simulink model "ModeAdjust"  (R2018b)
settings: Solver=FixedStepDiscrete  StartTime=0.0  StopTime=inf  FixedStep=0.01  RelTol=1e-3
undefined symbols (not defined in the file or in its folder): IfKeSMSbSeatMovBkRclnEnable_Val, IfKeSMSbSeatMovFrwdBkwdEnable_Val, IfKeSMSbSeatMovFtrstEnable_Val, IfKeSMSbSeatMovHdrstFrwdBkwdEnable_Val, IfKeSMSbSeatMovHdUpwdDnwdEnable_Val, IfKeSMSbSeatMovLgrstEnable_Val, IfKeSMSbSeatMovLtwdRtwdEnable_Val, IfVeSMSeStNumConfig, KeSMSbArmscreenMovEnable_Val, KeSMSbSeatMovLgrstExpdEnable_Val, KeSMSuFirstRwStBackPosDelta_Val, KeSMSuFirstRwStBackPosTolr_Val, KeSMSuFirstRwStCushFrntPosDelta_Val, KeSMSuFirstRwStCushFrntPosTolr_Val, KeSMSuFirstRwStCushRePosDelta_Val, KeSMSuFirstRwStCushRePosTolr_Val, KeSMSuFirstRwStFootrestPosDelta_Val, KeSMSuFirstRwStFootrestPosTolr_Val, KeSMSuFirstRwStFwdBkwdPosDelta_Val, KeSMSuFirstRwStFwdBkwdPosTolr_Val, KeSMSuMdMotFinshdTm_Val, KeSMSuMdRetryTm1_Val, KeSMSuModeReqDurgTm_Val, KeSMSuSecRwStArmTochPosDelta_Val, KeSMSuSecRwStArmTochPosTolr_Val, KeSMSuSecRwStBackPosDelta_Val, KeSMSuSecRwStBackPosTolr_Val, KeSMSuSecRwStFtrstUpwdDnwdPosDelta_Val, KeSMSuSecRwStFtrstUpwdDnwdPosTolr_Val, KeSMSuSecRwStFwdBkwdPosDelta_Val, KeSMSuSecRwStFwdBkwdPosTolr_Val, KeSMSuSecRwStHeadrestFwdBkwdPosDelta_Val, KeSMSuSecRwStHeadrestFwdBkwdPosTolr_Val, KeSMSuSecRwStHeadrestUpwdDwnwdPosDelta_Val, KeSMSuSecRwStHeadrestUpwdDwnwdPosTolr_Val, KeSMSuSecRwStLegrestInOutPosDelta_Val, KeSMSuSecRwStLegrestInOutPosTolr_Val, KeSMSuSecRwStLegrestUpwdDwnwdPosDelta_Val, KeSMSuSecRwStLegrestUpwdDwnwdPosTolr_Val, KeSMSuSecRwStLwdRwdPosDelta_Val, KeSMSuSecRwStLwdRwdPosTolr_Val, KeSMSuSecRwStVIPFtrstRefAngle_Val, KeSMSuThirdRwStFwdBkwdPosDelta_Val, KeSMSuThirdRwStFwdBkwdPosTolr_Val, KeSMSuThrdRwCushFoldPosDelta_Val, KeSMSuThrdRwCushFoldPosTolr_Val, KeSMSuThrdRwStBackPosDelta_Val, KeSMSuThrdRwStBackPosTolr_Val, KeSMSw4SLegrstCloseMdSecRwLtStFtrstUpwdDnwdPos_Val, KeSMSw4SLegrstCloseMdSecRwLtStFtrstUpwdDnwdPosMax_Val, KeSMSw4SLegrstCloseMdSecRwLtStFtrstUpwdDnwdPosMin_Val, KeSMSw4SLegrstCloseMdSecRwLtStLgrstOtwdInwdPos_Val, KeSMSw4SLegrstCloseMdSecRwLtStLgrstOtwdInwdPosMax_Val, KeSMSw4SLegrstCloseMdSecRwLtStLgrstOtwdInwdPosMin_Val, KeSMSw4SLegrstCloseMdSecRwLtStLgrstUpwdDnwdPos_Val, KeSMSw4SLegrstCloseMdSecRwLtStLgrstUpwdDnwdPosMax_Val, KeSMSw4SLegrstCloseMdSecRwLtStLgrstUpwdDnwdPosMin_Val, KeSMSw4SLegrstCloseMdSecRwRtStFtrstUpwdDnwdPos_Val, KeSMSw4SLegrstCloseMdSecRwRtStFtrstUpwdDnwdPosMax_Val, KeSMSw4SLegrstCloseMdSecRwRtStFtrstUpwdDnwdPosMin_Val ... (+1138)
libraries: Lib x401
(part 21 of 35)

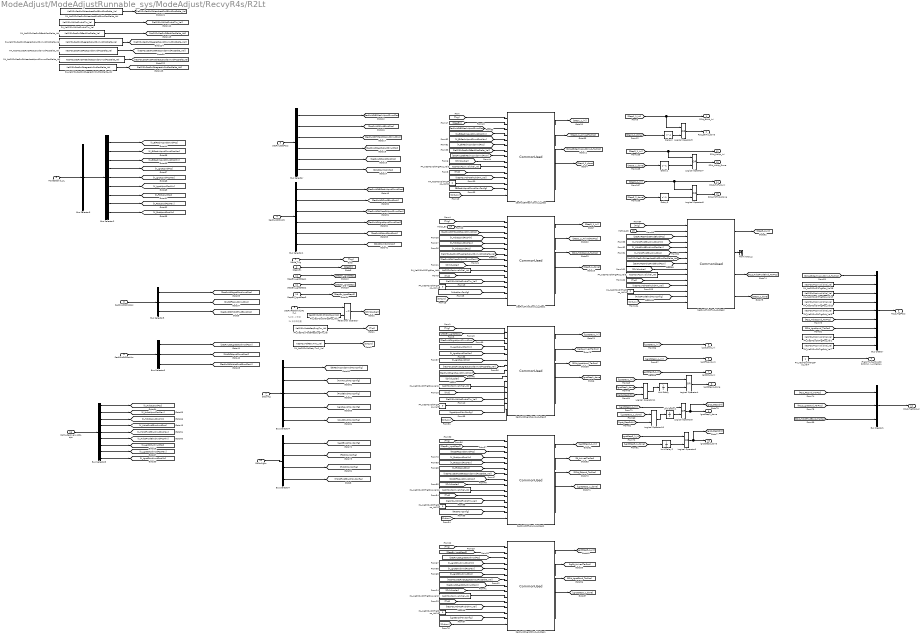
== system ModeAdjust/ModeAdjustRunnable_sys/ModeAdjust/RecvyR4s/R2Lt ==
  note: %1锁，2未锁
  note: 2L 扶手屏位置
  Mode_Trig : Inport
  Step1En : Inport  Port=2
  SecRwLtStsPoss : Inport  Port=3
  SecRwLtStPossV : Inport  Port=4
  SecRwRtStChldLkRsp_L : Inport  Port=5
  ModeStCalib_2L : Inport  Port=6
  StConfig : Inport  Port=7
  SecRwLtStsPoss4s : Inport  Port=8
  SecRwLtStPossV4s : Inport  Port=9
  StConfig4s : Inport  Port=10
  StepEn_LgrstStep1 : Inport  Port=11
  StepEn_LgrstStep2 : Inport  Port=12
  StepEn_LgrstStep3 : Inport  Port=13
  HdUp_En : Inport  Port=14
  HdFwd_En : Inport  Port=15
  Calib_Recovery4sRAdpt : Inport  Port=16
  Bus Creator : BusCreator  Inputs=9  OutDataTypeStr=Bus: SecRwRtSeatPos
  Bus Creator1 : BusCreator  Inputs=3
  Bus Selector : BusSelector  OutputSignals=IfVeSMSuSecRwRtStBkReclnUpwdDnwdPos_Val_read,IfVeSMSuSecRwRtStFrwdBkwdPos_Val_read,IfVeSMSuSecRwRtStHPassStUpwdDnwdPos_Val_read,IfVeSMSuSecRwRtStLgrstUpwdDnwdPos_Val_read,IfVeSMSuSecRwRtStLtwdRtwdPos_Val_read,SecRwRtStArmScrnPos_Val_read
  Bus Selector1 : BusSelector  OutputSignals=IfVeSMSuSecRwRtStBkReclnUpwdDnwdPosV_Val_read,IfVeSMSuSecRwRtStFrwdBkwdPosV_Val_read,IfVeSMSuSecRwRtStHPassStUpwdDnwdPosV_Val_read,IfVeSMSuSecRwRtStLgrstUpwdDnwdPosV_Val_read,IfVeSMSuSecRwRtStLtwdRtwdPosV_Val_read,SecRwRtStArmScrnPosV_Val_read
  Bus Selector2 : BusSelector  OutputSignals=BkReclnUpwdDnwdPos,BkReclnUpwdDnwdPosMax,BkReclnUpwdDnwdPosMin,LgrstUpwdPos,LgrstUpwdPosMax,LgrstUpwdPosMin,FtrstUpwdDnwdPos,FtrstUpwdDnwdPosMax,FtrstUpwdDnwdPosMin
  Bus Selector3 : BusSelector  OutputSignals=RecvyRSecRwRtSt
  Bus Selector4 : BusSelector  OutputSignals=BkReclnUpwdDnwdMovConfig,ArmTouchMovConfig,FrwdBkwdMovConfig,LgrstUpwdMovConfig,LtwdRtwdMovConfig
  Bus Selector5 : BusSelector  OutputSignals=IfVeSMSuSecRwRtStLgrstOtwdInwdPos_Val_read,IfVeSMSuRrRtStFtUpwdDnwdPos_Val_read,IfVeSMSuSecRwRtStHdrstFrwdBkwdPos_Val_read
  Bus Selector6 : BusSelector  OutputSignals=IfVeSMSuSecRwRtStLgrstOtwdInwdPosV_Val_read,IfVeSMSuRrRtStFtUpwdDnwdPosV_Val_read,IfVeSMSuSecRwRtStHdrstFrwdBkwdPosV_Val_read
  Bus Selector7 : BusSelector  OutputSignals=LgrstExpdMovConfig,FtrstMovConfig,HdrstUpwdDnwdMovConfig,HdrstFrwdBkwdMovConfig
  Bus Selector8 : BusSelector  OutputSignals=HdrstUpwdDnwdPos,HdrstUpwdDnwdPosMax,HdrstUpwdDnwdPosMin,HdrstFrwdBkwdnwdPos,HdrstFrwdBkwdnwdPosMax,HdrstFrwdBkwdnwdPosMin,LgrstOtwdInwdPos,LgrstOtwdInwdPosMax,LgrstOtwdInwdPosMin
  Delay1 : Delay  DelayLength=1
  Delay2 : Delay  DelayLength=1
  Delay3 : Delay  DelayLength=1
  Logical Operator10 : Logic  AllPortsSameDT=off  OutDataTypeStr=boolean
  Logical Operator11 : Logic  AllPortsSameDT=off  OutDataTypeStr=boolean
  Logical Operator{3..8} (6 alike) : Logic  Operator=OR  AllPortsSameDT=off  OutDataTypeStr=boolean
  PA_KeSMSuMdMotFinshdTm_Val : Constant  Value=KeSMSuMdMotFinshdTm_Val
  PA_KeSMSuMdRetryTm1_Val : Constant  Value=KeSMSuMdRetryTm1_Val
  PA_KeSMSuModeReqDurgTm_Val : Constant  Value=KeSMSuModeReqDurgTm_Val
  PA_KeSMSuSecRwStBackPosDelta_Val : Constant  Value=KeSMSuSecRwStBackPosDelta_Val
  PA_KeSMSuSecRwStFtrstUpwdDnwdPosDelta_Val : Constant  Value=KeSMSuSecRwStFtrstUpwdDnwdPosDelta_Val
  PA_KeSMSuSecRwStHeadrestFwdBkwdPosDelta_Val : Constant  Value=KeSMSuSecRwStHeadrestFwdBkwdPosDelta_Val
  PA_KeSMSuSecRwStHeadrestUpwdDwnwdPosDelta_Val : Constant  Value=KeSMSuSecRwStHeadrestUpwdDwnwdPosDelta_Val
  PA_KeSMSuSecRwStLegrestInOutPosDelta_Val : Constant  Value=KeSMSuSecRwStLegrestInOutPosDelta_Val
  PA_KeSMSuSecRwStLegrestUpwdDwnwdPosDelta_Val : Constant  Value=KeSMSuSecRwStLegrestUpwdDwnwdPosDelta_Val
  PA_KeSMSwDltTrgtPos_Val{1,3,5..8,12..13,16,18..20} (12 alike) : Constant  Value=KeSMSwPosInvalidVal_Val
  PA_KeSMSwDltTrgtPos_Val{9..11,15,22,30} (6 alike) : Constant  Value=0  OutDataTypeStr=boolean
  PA_KeSMSwDltTrgtPos_Val2 : Constant  Value=SeatChldLkSt.ChldLkSt_Unlock
  PA_KeSMSwDltTrgtPos_Val4 : Constant  OutDataTypeStr=boolean
  Relational Operator : RelationalOperator  Operator=~=  OutDataTypeStr=boolean  RndMeth=Simplest
  SecRwLtBkRecInUpwd_Lt_Step : Lib/CommonUsed  SystemSampleTime=-1
  SecRwLtHdrstFwd_Lt_Step2 : Lib/CommonUsed  SystemSampleTime=-1
  SecRwLtHdrstUpwd_Lt_Step1 : Lib/CommonUsed  SystemSampleTime=-1
  SecRwLtStFtUpwd_Lt_Step2 : Lib/CommonUsed  SystemSampleTime=-1
  SecRwLtStLgrstOtwd_Lt_Step1 : Lib/CommonUsed  SystemSampleTime=-1
  SecRwLtStLgrstUpwd_Lt_Step3 : Lib/CommonUsed  SystemSampleTime=-1
  Terminator_2 : Terminator
  Unit Delay : UnitDelay  SampleTime=-1
  Unit Delay1 : UnitDelay  SampleTime=-1
  Unit Delay2 : UnitDelay  SampleTime=-1
  R2Lt_BkHd_Ini : Outport
  R2Lt_BkHd_done : Outport  Port=2
  R2Lt_TrgtPoss : Outport  Port=3  VectorParamsAs1DForOutWhenUnconnected=on
  IfVeSMSuSecRwLtStRclCmdSrv_Val_writeRaw : Outport  Port=4
  lgrstUpwd_ini : Outport  Port=5  VectorParamsAs1DForOutWhenUnconnected=on
  lgrstFtUpwd_ini : Outport  Port=6  VectorParamsAs1DForOutWhenUnconnected=on
  lgrstOtwd_ini : Outport  Port=7  VectorParamsAs1DForOutWhenUnconnected=on
  lgrstStep1_done : Outport  Port=8  VectorParamsAs1DForOutWhenUnconnected=on
  lgrstStep2_done : Outport  Port=9  VectorParamsAs1DForOutWhenUnconnected=on
  lgrstStep3_done : Outport  Port=10  VectorParamsAs1DForOutWhenUnconnected=on
  R2Lt_TrgtPoss_2 : Outport  Port=11  VectorParamsAs1DForOutWhenUnconnected=on
  R2Lt_HdUp_Ini : Outport  Port=12
  R2Lt_HdUp_Done : Outport  Port=13
  R2Lt_HdFwd_Ini : Outport  Port=14
  R2Lt_HdFwd_Done : Outport  Port=15
  wires:
  Logical Operator11/1 -> Unit Delay/1
  [lgrst_Step2chk] -> Logical Operator11/2
  [lgrstStep1_done] -> Logical Operator11/1
  [lgrst_Step3chk] -> Logical Operator10/2
  Logical Operator10/1 -> Unit Delay1/1
  [LgrstStep2_1_done] -> Logical Operator10/1
  [R2Lt_LgrstOtwd_TarPos] -> Bus Creator1/2  "SecRwRtStLgrstOtwdInwdTrgtPos"
  [R2Lt_FtUpwd_TarPos] -> Bus Creator1/1  "RrRtStFtUpwdDnwdTrgtPos"
  Bus Creator1/1 -> R2Lt_TrgtPoss_2/1
  [LgrstStep3_1_ini] -> Logical Operator6/1
  [LgrstStep2_1_ini] -> Logical Operator5/1
  [LgrstStep3_1_done] -> Unit Delay2/1
  Unit Delay2/1 -> Logical Operator6/2
  Logical Operator6/1 -> lgrstStep3_done/1, [lgrst_Step3chk]
  Unit Delay1/1 -> Logical Operator5/2
  Logical Operator5/1 -> lgrstStep2_done/1, [lgrst_Step2chk]
  Unit Delay/1 -> Logical Operator4/2
  [lgrstStep1_ini] -> Logical Operator4/1
  Logical Operator4/1 -> lgrstStep1_done/1
  StepEn_LgrstStep3/1 -> [StepEn_LgrstStep3]
  StepEn_LgrstStep2/1 -> [StepEn_LgrstStep2]
  StepEn_LgrstStep1/1 -> [StepEn_LgrstStep1]
  [LgrstStep3_1_ini] -> lgrstOtwd_ini/1
  [LgrstStep2_1_ini] -> lgrstFtUpwd_ini/1
  [lgrstStep1_ini] -> lgrstUpwd_ini/1
  PA_KeSMSwDltTrgtPos_Val30/1 -> SecRwLtBkRecInUpwd_Lt_Step/13
  Bus Selector7/3 -> [HdrstMovConfig]  "<HdrstUpwdDnwdMovConfig>"
  Bus Selector7/2 -> [FtrstMovConfig]  "<FtrstMovConfig>"
  Bus Selector7/1 -> [LgrstExpdMovConfig]  "<LgrstExpdMovConfig>"
  StConfig4s/1 -> Bus Selector7/1
  [FtrstMovConfig] -> SecRwLtStFtUpwd_Lt_Step2/14
  PA_KeSMSwDltTrgtPos_Val22/1 -> SecRwLtStFtUpwd_Lt_Step2/13
  [KeSMSuMdMotFinshdTm_Val] -> SecRwLtStFtUpwd_Lt_Step2/12
  SecRwLtStFtUpwd_Lt_Step2/4 -> [LgrstStep2_1_done]
  SecRwLtStFtUpwd_Lt_Step2/3 -> [R2Lt_FtUpwd_TarPos]
  SecRwLtStFtUpwd_Lt_Step2/2 -> [Ft_ArrivedTarPos]
  [Tick] -> SecRwLtStFtUpwd_Lt_Step2/11
  PA_KeSMSwDltTrgtPos_Val16/1 -> SecRwLtStFtUpwd_Lt_Step2/10
  [ChildLocker] -> SecRwLtStFtUpwd_Lt_Step2/9
  [RrLtStFtUpwdDnwdPosV] -> SecRwLtStFtUpwd_Lt_Step2/8
  [KeSMSuSecRwStFtrstUpwdDnwdPosDelta_Val] -> SecRwLtStFtUpwd_Lt_Step2/7
  [RrLtStFtUpwdDnwdPos] -> SecRwLtStFtUpwd_Lt_Step2/3
  [K_FtrstUpwdPos] -> SecRwLtStFtUpwd_Lt_Step2/6
  [K_FtrstUpwdPosMax] -> SecRwLtStFtUpwd_Lt_Step2/5
  [K_FtrstUpwdPosMin] -> SecRwLtStFtUpwd_Lt_Step2/4
  [StepEn_LgrstStep2] -> SecRwLtStFtUpwd_Lt_Step2/2
  [Trig] -> SecRwLtStFtUpwd_Lt_Step2/1
  SecRwLtStFtUpwd_Lt_Step2/1 -> [LgrstStep2_1_ini]
  SecRwLtStLgrstOtwd_Lt_Step1/1 -> [LgrstStep3_1_ini]
  [Trig] -> SecRwLtStLgrstOtwd_Lt_Step1/1
  [StepEn_LgrstStep3] -> SecRwLtStLgrstOtwd_Lt_Step1/2
  [K_LgrstOtwdInwdPosMin] -> SecRwLtStLgrstOtwd_Lt_Step1/4
  [K_LgrstOtwdInwdPosMax] -> SecRwLtStLgrstOtwd_Lt_Step1/5
  [K_LgrstOtwdInwdPos] -> SecRwLtStLgrstOtwd_Lt_Step1/6
  [SecRwLtStLgrstOtwdInwdPos] -> SecRwLtStLgrstOtwd_Lt_Step1/3
  [KeSMSuSecRwStLegrestInOutPosDelta_Val] -> SecRwLtStLgrstOtwd_Lt_Step1/7
  [SecRwLtStLgrstOtwdInwdPosV] -> SecRwLtStLgrstOtwd_Lt_Step1/8
  [ChildLocker] -> SecRwLtStLgrstOtwd_Lt_Step1/9
  PA_KeSMSwDltTrgtPos_Val13/1 -> SecRwLtStLgrstOtwd_Lt_Step1/10
  [Tick] -> SecRwLtStLgrstOtwd_Lt_Step1/11
  SecRwLtStLgrstOtwd_Lt_Step1/2 -> [LgOt_ArrivedTarPos]
  SecRwLtStLgrstOtwd_Lt_Step1/3 -> [R2Lt_LgrstOtwd_TarPos]
  SecRwLtStLgrstOtwd_Lt_Step1/4 -> [LgrstStep3_1_done]
  [KeSMSuMdMotFinshdTm_Val] -> SecRwLtStLgrstOtwd_Lt_Step1/12
  PA_KeSMSwDltTrgtPos_Val15/1 -> SecRwLtStLgrstOtwd_Lt_Step1/13
  [LgrstExpdMovConfig] -> SecRwLtStLgrstOtwd_Lt_Step1/14
  Bus Selector6/2 -> [RrLtStFtUpwdDnwdPosV]  "<IfVeSMSuRrRtStFtUpwdDnwdPosV_Val_read>"
  Bus Selector6/1 -> [SecRwLtStLgrstOtwdInwdPosV]  "<IfVeSMSuSecRwRtStLgrstOtwdInwdPosV_Val_read>"
  Bus Selector5/2 -> [RrLtStFtUpwdDnwdPos]  "<IfVeSMSuRrRtStFtUpwdDnwdPos_Val_read>"
  Bus Selector5/1 -> [SecRwLtStLgrstOtwdInwdPos]  "<IfVeSMSuSecRwRtStLgrstOtwdInwdPos_Val_read>"
  SecRwLtStPossV4s/1 -> Bus Selector6/1
  SecRwLtStsPoss4s/1 -> Bus Selector5/1
  PA_KeSMSuSecRwStLegrestInOutPosDelta_Val/1 -> [KeSMSuSecRwStLegrestInOutPosDelta_Val]
  PA_KeSMSuSecRwStHeadrestUpwdDwnwdPosDelta_Val/1 -> [KeSMSuSecRwStHeadrestUpwdDwnwdPosDelta_Val]
  PA_KeSMSuSecRwStFtrstUpwdDnwdPosDelta_Val/1 -> [KeSMSuSecRwStFtrstUpwdDnwdPosDelta_Val]
  Bus Selector2/7 -> [K_FtrstUpwdPos]  "<FtrstUpwdDnwdPos>"
  Bus Selector2/8 -> [K_FtrstUpwdPosMax]  "<FtrstUpwdDnwdPosMax>"
  Bus Selector2/9 -> [K_FtrstUpwdPosMin]  "<FtrstUpwdDnwdPosMin>"
  SecRwLtHdrstUpwd_Lt_Step1/1 -> [Step3_1_ini]
  [Trig] -> SecRwLtHdrstUpwd_Lt_Step1/1
  HdUp_En/1 -> SecRwLtHdrstUpwd_Lt_Step1/2
  [K_HdrstUpwdPosMin] -> SecRwLtHdrstUpwd_Lt_Step1/4
  [K_HdrstUpwdPosMax] -> SecRwLtHdrstUpwd_Lt_Step1/5
  [K_HdrstUpwdPos] -> SecRwLtHdrstUpwd_Lt_Step1/6
  [SecRwLtStHPassStUpwdDnwdPos] -> SecRwLtHdrstUpwd_Lt_Step1/3
  [KeSMSuSecRwStHeadrestUpwdDwnwdPosDelta_Val] -> SecRwLtHdrstUpwd_Lt_Step1/7
  [SecRwLtStHPassStUpwdDnwdPosV] -> SecRwLtHdrstUpwd_Lt_Step1/8
  [ChildLocker] -> SecRwLtHdrstUpwd_Lt_Step1/9
  PA_KeSMSwDltTrgtPos_Val6/1 -> SecRwLtHdrstUpwd_Lt_Step1/10
  [Tick] -> SecRwLtHdrstUpwd_Lt_Step1/11
  SecRwLtHdrstUpwd_Lt_Step1/2 -> [Step1_2_ArrivedTarPos]
  SecRwLtHdrstUpwd_Lt_Step1/3 -> [R2Lt_HdrstUpwd_TarPos]
  SecRwLtHdrstUpwd_Lt_Step1/4 -> [Step3_1_done]
  [KeSMSuMdMotFinshdTm_Val] -> SecRwLtHdrstUpwd_Lt_Step1/12
  PA_KeSMSwDltTrgtPos_Val11/1 -> SecRwLtHdrstUpwd_Lt_Step1/13
  [HdrstMovConfig] -> SecRwLtHdrstUpwd_Lt_Step1/14
  [BkReclnUpwdDnwdMovConfig] -> SecRwLtBkRecInUpwd_Lt_Step/14
  [LgrstUpwdMovConfig] -> SecRwLtStLgrstUpwd_Lt_Step3/14
  PA_KeSMSwDltTrgtPos_Val9/1 -> SecRwLtStLgrstUpwd_Lt_Step3/13
  Bus Selector4/1 -> [BkReclnUpwdDnwdMovConfig]  "<BkReclnUpwdDnwdMovConfig>"
  Bus Selector4/2 -> [ArmTouchMovConfig]  "<ArmTouchMovConfig>"
  Bus Selector4/4 -> [LgrstUpwdMovConfig]  "<LgrstUpwdMovConfig>"
  Bus Selector4/5 -> [LtwdRtwdMovConfig]  "<LtwdRtwdMovConfig>"
  Bus Selector4/3 -> [FrwdBkwdMovConfig]  "<FrwdBkwdMovConfig>"
  StConfig/1 -> Bus Selector4/1
  ModeStCalib_2L/1 -> Bus Selector3/1
  Bus Selector2/3 -> [K_BkReclnUpwdDnwdPosMin]  "<BkReclnUpwdDnwdPosMin>"
  Bus Selector3/1 -> Bus Selector2/1  "<RecvyRSecRwRtSt>"
  Bus Selector2/2 -> [K_BkReclnUpwdDnwdPosMax]  "<BkReclnUpwdDnwdPosMax>"
  Bus Selector2/1 -> [K_BkReclnUpwdDnwdPos]  "<BkReclnUpwdDnwdPos>"
  Bus Selector2/5 -> [K_LgrstUpwdPosMax]  "<LgrstUpwdPosMax>"
  Bus Selector2/4 -> [K_LgrstUpwdPos]  "<LgrstUpwdPos>"
  Bus Selector2/6 -> [K_LgrstUpwdPosMin]  "<LgrstUpwdPosMin>"
  Bus Selector1/6 -> [R2LtStArmScrnPosV]  "<SecRwRtStArmScrnPosV_Val_read>"
  Bus Selector/6 -> [R2LtStArmScrnPos]  "<SecRwRtStArmScrnPos_Val_read>"
  [KeSMSuMdMotFinshdTm_Val] -> SecRwLtStLgrstUpwd_Lt_Step3/12
  [KeSMSuMdMotFinshdTm_Val] -> SecRwLtBkRecInUpwd_Lt_Step/12
  PA_KeSMSuMdMotFinshdTm_Val/1 -> [KeSMSuMdMotFinshdTm_Val]
  PA_KeSMSuSecRwStLegrestUpwdDwnwdPosDelta_Val/1 -> [KeSMSuSecRwStLegrestUpwdDwnwdPosDelta_Val]
  PA_KeSMSuSecRwStBackPosDelta_Val/1 -> [KeSMSuSecRwStBackPosDelta_Val]
  PA_KeSMSwDltTrgtPos_Val7/1 -> Bus Creator/9  "SecRwRtStArmScrnTrgtPos"
  PA_KeSMSuModeReqDurgTm_Val/1 -> [Tick]
  Delay2/1 -> Logical Operator3/2
  [Step1_1_done] -> Delay2/1
  [StepEn] -> SecRwLtBkRecInUpwd_Lt_Step/2
  Logical Operator3/1 -> R2Lt_BkHd_done/1
  Step1En/1 -> [StepEn]
  PA_KeSMSwDltTrgtPos_Val20/1 -> Bus Creator/4  "SecRwRtStCshnRrUpwdDnwdTrgtPos"
  PA_KeSMSwDltTrgtPos_Val8/1 -> Bus Creator/5  "SecRwRtStFrwdBkwdTrgtPos"
  [R2Lt_BkReclnUpwdDnwd_TarPos] -> Bus Creator/1  "SecRwRtStBkReclnUpwdDnwdTrgtPos"
  PA_KeSMSwDltTrgtPos_Val18/1 -> Bus Creator/2  "SecRwRtStBlstOtwdInwdTrgtPos"
  PA_KeSMSwDltTrgtPos_Val1/1 -> Bus Creator/8  "SecRwRtStLtwdRtwdTrgtPos"
  PA_KeSMSwDltTrgtPos_Val19/1 -> Bus Creator/3  "SecRwRtStCshnFrntUpwdDnwdTrgtPos"
  [R2Lt_LgrstUpwd_TarPos] -> Bus Creator/7  "SecRwRtStLgrstUpwdDnwdTrgtPos"
  Bus Creator/1 -> R2Lt_TrgtPoss/1
  [R2Lt_HdrstUpwd_TarPos] -> Bus Creator/6  "SecRwRtStHdrstUpwdDnwdTrgtPos"
  SecRwLtBkRecInUpwd_Lt_Step/1 -> [Step1_1_ini]
  SecRwLtStLgrstUpwd_Lt_Step3/4 -> [lgrstStep1_done]
  SecRwLtStLgrstUpwd_Lt_Step3/3 -> [R2Lt_LgrstUpwd_TarPos]
  SecRwLtStLgrstUpwd_Lt_Step3/2 -> [lgrst_ArrivedTarPos]
  [Tick] -> SecRwLtStLgrstUpwd_Lt_Step3/11
  PA_KeSMSwDltTrgtPos_Val12/1 -> SecRwLtStLgrstUpwd_Lt_Step3/10
  [ChildLocker] -> SecRwLtStLgrstUpwd_Lt_Step3/9
  [SecRwLtStLgrstUpwdDnwdPosV] -> SecRwLtStLgrstUpwd_Lt_Step3/8
  [KeSMSuSecRwStLegrestUpwdDwnwdPosDelta_Val] -> SecRwLtStLgrstUpwd_Lt_Step3/7
  [SecRwLtStBkReclnUpwdDnwdPosV] -> SecRwLtBkRecInUpwd_Lt_Step/8
  [SecRwLtStLgrstUpwdDnwdPos] -> SecRwLtStLgrstUpwd_Lt_Step3/3
  [K_LgrstUpwdPos] -> SecRwLtStLgrstUpwd_Lt_Step3/6
  [K_LgrstUpwdPosMax] -> SecRwLtStLgrstUpwd_Lt_Step3/5
  [K_LgrstUpwdPosMin] -> SecRwLtStLgrstUpwd_Lt_Step3/4
  [StepEn_LgrstStep1] -> SecRwLtStLgrstUpwd_Lt_Step3/2
  [Trig] -> SecRwLtStLgrstUpwd_Lt_Step3/1
  Relational Operator/1 -> [ChildLocker]
  PA_KeSMSwDltTrgtPos_Val2/1 -> Relational Operator/2
  SecRwRtStChldLkRsp_L/1 -> Relational Operator/1
  Bus Selector/1 -> [SecRwLtStBkReclnUpwdDnwdPos]  "<IfVeSMSuSecRwRtStBkReclnUpwdDnwdPos_Val_read>"
  Bus Selector1/2 -> [SecRwLtStFrwdBkwdPosV]  "<IfVeSMSuSecRwRtStFrwdBkwdPosV_Val_read>"
  Bus Selector1/1 -> [SecRwLtStBkReclnUpwdDnwdPosV]  "<IfVeSMSuSecRwRtStBkReclnUpwdDnwdPosV_Val_read>"
  Bus Selector/2 -> [SecRwLtStFrwdBkwdPos]  "<IfVeSMSuSecRwRtStFrwdBkwdPos_Val_read>"
  Bus Selector/4 -> [SecRwLtStLgrstUpwdDnwdPos]  "<IfVeSMSuSecRwRtStLgrstUpwdDnwdPos_Val_read>"
  Bus Selector1/5 -> [SecRwLtStLtwdRtwdPosV]  "<IfVeSMSuSecRwRtStLtwdRtwdPosV_Val_read>"
  Bus Selector/3 -> [SecRwLtStHPassStUpwdDnwdPos]  "<IfVeSMSuSecRwRtStHPassStUpwdDnwdPos_Val_read>"
  SecRwLtStPossV/1 -> Bus Selector1/1
  Bus Selector1/4 -> [SecRwLtStLgrstUpwdDnwdPosV]  "<IfVeSMSuSecRwRtStLgrstUpwdDnwdPosV_Val_read>"
  SecRwLtStsPoss/1 -> Bus Selector/1
  Bus Selector/5 -> [SecRwLtStLtwdRtwdPos]  "<IfVeSMSuSecRwRtStLtwdRtwdPos_Val_read>"
  Bus Selector1/3 -> [SecRwLtStHPassStUpwdDnwdPosV]  "<IfVeSMSuSecRwRtStHPassStUpwdDnwdPosV_Val_read>"
  [Tick] -> SecRwLtBkRecInUpwd_Lt_Step/11
  [ChildLocker] -> SecRwLtBkRecInUpwd_Lt_Step/9
  SecRwLtBkRecInUpwd_Lt_Step/3 -> [R2Lt_BkReclnUpwdDnwd_TarPos]
  PA_KeSMSwDltTrgtPos_Val3/1 -> SecRwLtBkRecInUpwd_Lt_Step/10
  [K_BkReclnUpwdDnwdPos] -> SecRwLtBkRecInUpwd_Lt_Step/6
  [SecRwLtStBkReclnUpwdDnwdPos] -> SecRwLtBkRecInUpwd_Lt_Step/3
  SecRwLtBkRecInUpwd_Lt_Step/2 -> [Step1_1_ArrivedTarPos]
  [K_BkReclnUpwdDnwdPosMin] -> SecRwLtBkRecInUpwd_Lt_Step/4
  [KeSMSuSecRwStBackPosDelta_Val] -> SecRwLtBkRecInUpwd_Lt_Step/7
  Mode_Trig/1 -> [Trig]
  [Trig] -> SecRwLtBkRecInUpwd_Lt_Step/1
  [K_BkReclnUpwdDnwdPosMax] -> SecRwLtBkRecInUpwd_Lt_Step/5
  [Step1_1_ini] -> R2Lt_BkHd_Ini/1, Logical Operator3/1
  SecRwLtStLgrstUpwd_Lt_Step3/1 -> [lgrstStep1_ini]
  SecRwLtBkRecInUpwd_Lt_Step/4 -> [Step1_1_done]
  PA_KeSMSwDltTrgtPos_Val4/1 -> IfVeSMSuSecRwLtStRclCmdSrv_Val_writeRaw/1
  [CntLow] -> SecRwLtBkRecInUpwd_Lt_Step/15
  [CntLow] -> SecRwLtHdrstUpwd_Lt_Step1/15
  [CntLow] -> SecRwLtStFtUpwd_Lt_Step2/15
  [CntLow] -> SecRwLtStLgrstOtwd_Lt_Step1/15
  [CntLow] -> SecRwLtStLgrstUpwd_Lt_Step3/15
  PA_KeSMSuMdRetryTm1_Val/1 -> [CntLow]
  [R2Lt_HdrstFrwdBkwd_TarPos] -> Bus Creator1/3  "SecRwRtStHdrstFrwdBkwdTrgtPos"
  Bus Selector7/4 -> [HdrstFrwdBkwdMovConfig]  "<HdrstFrwdBkwdMovConfig>"
  Bus Selector5/3 -> [SecRwRtStHdrstFrwdBkwdPos]  "<IfVeSMSuSecRwRtStHdrstFrwdBkwdPos_Val_read>"
  Bus Selector6/3 -> [SecRwRtStHdrstFrwdBkwdPosV]  "<IfVeSMSuSecRwRtStHdrstFrwdBkwdPosV_Val_read>"
  PA_KeSMSuSecRwStHeadrestFwdBkwdPosDelta_Val/1 -> [KeSMSuSecRwStHeadrestFwdBkwdPosDelta_Val]
  [CntLow] -> SecRwLtHdrstFwd_Lt_Step2/15
  [K_HdrstFrwdBkwdnwdPosMax] -> SecRwLtHdrstFwd_Lt_Step2/5
  [HdrstFrwdBkwdMovConfig] -> SecRwLtHdrstFwd_Lt_Step2/14
  [SecRwRtStHdrstFrwdBkwdPosV] -> SecRwLtHdrstFwd_Lt_Step2/8
  [KeSMSuSecRwStHeadrestFwdBkwdPosDelta_Val] -> SecRwLtHdrstFwd_Lt_Step2/7
  [SecRwRtStHdrstFrwdBkwdPos] -> SecRwLtHdrstFwd_Lt_Step2/3
  [K_HdrstFrwdBkwdnwdPos] -> SecRwLtHdrstFwd_Lt_Step2/6
  PA_KeSMSwDltTrgtPos_Val5/1 -> SecRwLtHdrstFwd_Lt_Step2/10
  SecRwLtHdrstFwd_Lt_Step2/3 -> [R2Lt_HdrstFrwdBkwd_TarPos]
  [ChildLocker] -> SecRwLtHdrstFwd_Lt_Step2/9
  SecRwLtHdrstFwd_Lt_Step2/1 -> [Step3_2_ini]
  [Tick] -> SecRwLtHdrstFwd_Lt_Step2/11
  SecRwLtHdrstFwd_Lt_Step2/2 -> Terminator_2/1
  [KeSMSuMdMotFinshdTm_Val] -> SecRwLtHdrstFwd_Lt_Step2/12
  HdFwd_En/1 -> SecRwLtHdrstFwd_Lt_Step2/2
  PA_KeSMSwDltTrgtPos_Val10/1 -> SecRwLtHdrstFwd_Lt_Step2/13
  [K_HdrstFrwdBkwdnwdPosMin] -> SecRwLtHdrstFwd_Lt_Step2/4
  [Trig] -> SecRwLtHdrstFwd_Lt_Step2/1
  SecRwLtHdrstFwd_Lt_Step2/4 -> [Step3_2_done]
  Logical Operator8/1 -> R2Lt_HdFwd_Done/1
  [Step3_2_done] -> Delay3/1
  [Step3_1_done] -> Delay1/1
  Delay3/1 -> Logical Operator8/2
  [Step3_2_ini] -> Logical Operator8/1, R2Lt_HdFwd_Ini/1
  Delay1/1 -> Logical Operator7/2
  Logical Operator7/1 -> R2Lt_HdUp_Done/1
  [Step3_1_ini] -> Logical Operator7/1, R2Lt_HdUp_Ini/1
  Bus Selector8/3 -> [K_HdrstUpwdPosMin]  "<HdrstUpwdDnwdPosMin>"
  Bus Selector8/2 -> [K_HdrstUpwdPosMax]  "<HdrstUpwdDnwdPosMax>"
  Calib_Recovery4sRAdpt/1 -> Bus Selector8/1
  Bus Selector8/1 -> [K_HdrstUpwdPos]  "<HdrstUpwdDnwdPos>"
  Bus Selector8/4 -> [K_HdrstFrwdBkwdnwdPos]  "<HdrstFrwdBkwdnwdPos>"
  Bus Selector8/5 -> [K_HdrstFrwdBkwdnwdPosMax]  "<HdrstFrwdBkwdnwdPosMax>"
  Bus Selector8/6 -> [K_HdrstFrwdBkwdnwdPosMin]  "<HdrstFrwdBkwdnwdPosMin>"
  Bus Selector8/7 -> [K_LgrstOtwdInwdPos]  "<LgrstOtwdInwdPos>"
  Bus Selector8/8 -> [K_LgrstOtwdInwdPosMax]  "<LgrstOtwdInwdPosMax>"
  Bus Selector8/9 -> [K_LgrstOtwdInwdPosMin]  "<LgrstOtwdInwdPosMin>"

== system ModeAdjust/ModeAdjustRunnable_sys/ModeAdjust/VIPL/Drv ==
  note: %1锁，2未锁
  Mode_Trig : Inport
  Step1En : Inport  Port=2
  DrvCurPos : Inport  Port=3
  DrvCurPosV : Inport  Port=4
  ModeStCalib_Drv : Inport  Port=5
  StConfig : Inport  Port=6
  SecRwRtStChldLkRsp_L : Inport  Port=7
  isSeatOccupied : Inport  Port=8
  Drv_FtUpwdDnwdPosTrgt : Inport  Port=9
  Bus Creator : BusCreator  Inputs=8  OutDataTypeStr=Bus: DrvSeatPos
  Bus Selector : BusSelector  OutputSignals=IfVeSMSuDrvStFtUpwdDnwdPos_Val_read,IfVeSMSuDrvStBkReclnUpwdDnwdPos_Val_read,IfVeSMSuDrvStCshnFrntUpwdDnwdPos_Val_read,IfVeSMSuDrvStCshnRrUpwdDnwdPos_Val_read,IfVeSMSuDrvStFrwdBkwdPos_Val_read
  Bus Selector1 : BusSelector  OutputSignals=IfVeSMSuDrvStFtUpwdDnwdPosV_Val_read,IfVeSMSuDrvStBkReclnUpwdDnwdPosV_Val_read,IfVeSMSuDrvStCshnFrntUpwdDnwdPosV_Val_read,IfVeSMSuDrvStCshnRrUpwdDnwdPosV_Val_read,IfVeSMSuDrvStFrwdBkwdPosV_Val_read
  Bus Selector2 : BusSelector  OutputSignals=BkReclnUpwdDnwdPos,BkReclnUpwdDnwdPosMax,BkReclnUpwdDnwdPosMin,FrwdBkwdPos,FrwdBkwdPosMax,FrwdBkwdPosMin,FtUpwdDnwdPos,FtUpwdDnwdPosMax,FtUpwdDnwdPosMin
  Bus Selector3 : BusSelector  OutputSignals=VIPDrvSt
  Bus Selector4 : BusSelector  OutputSignals=BkReclnUpwdDnwdMovConfig,FrwdBkwdMovConfig,FtUpwdDnwdMovConfig
  DrvSt_DrvStFtUpwdDnwd_Step1 : Lib/CommonUsed  SystemSampleTime=-1
  Logical Operator : Logic  Operator=OR  AllPortsSameDT=off  OutDataTypeStr=boolean
  Logical Operator10 : Logic  Operator=OR  AllPortsSameDT=off  OutDataTypeStr=boolean
  PA_KeSMSuFirstRwStBackPosDelta_Val : Constant  Value=KeSMSuFirstRwStBackPosDelta_Val
  PA_KeSMSuFirstRwStFootrestPosDelta_Val : Constant  Value=KeSMSuFirstRwStFootrestPosDelta_Val
  PA_KeSMSuFirstRwStFwdBkwdPosDelta_Val : Constant  Value=KeSMSuFirstRwStFwdBkwdPosDelta_Val
  PA_KeSMSuMdMotFinshdTm_Val : Constant  Value=KeSMSuMdMotFinshdTm_Val
  PA_KeSMSuMdRetryTm1_Val : Constant  Value=KeSMSuMdRetryTm1_Val
  PA_KeSMSuModeReqDurgTm_Val : Constant  Value=KeSMSuModeReqDurgTm_Val
  PA_KeSMSwDltTrgtPos_Val{1..3,10,13..16} (8 alike) : Constant  Value=KeSMSwPosInvalidVal_Val
  PA_KeSMSwDltTrgtPos_Val4 : Constant  Value=SeatChldLkSt.ChldLkSt_Unlock
  PA_KeSMSwDltTrgtPos_Val5 : Constant  Value=0  OutDataTypeStr=boolean
  PA_KeSMSwDltTrgtPos_Val7 : Constant  OutDataTypeStr=boolean
  Relational Operator : RelationalOperator  Operator=~=  OutDataTypeStr=boolean  RndMeth=Simplest
  Unit Delay : UnitDelay  SampleTime=-1
  DrvSt_Step1_ini : Outport
  DrvSt_Step1_done : Outport  Port=2
  Recv_DrvStTrgtPoss : Outport  Port=3  VectorParamsAs1DForOutWhenUnconnected=on
  IfVeSMSuDrvStRclCmdSrv_Val_writeRaw : Outport  Port=4
  wires:
  DrvSt_DrvStFtUpwdDnwd_Step1/4 -> [Step1done_2]
  DrvSt_DrvStFtUpwdDnwd_Step1/3 -> [DrvSt_FtUpwdDnwd_TarPos]
  DrvSt_DrvStFtUpwdDnwd_Step1/2 -> [Step1_2_ArrivedTarPos]
  DrvSt_DrvStFtUpwdDnwd_Step1/1 -> [FtUpwdDnwd_Step1_ini]
  [Tick] -> DrvSt_DrvStFtUpwdDnwd_Step1/11
  PA_KeSMSwDltTrgtPos_Val1/1 -> DrvSt_DrvStFtUpwdDnwd_Step1/10
  [ChildLocker] -> DrvSt_DrvStFtUpwdDnwd_Step1/9
  [DrvStFtUpwdDnwdPosV] -> DrvSt_DrvStFtUpwdDnwd_Step1/8
  [KeSMSuFirstRwStFootrestPosDelta_Val] -> DrvSt_DrvStFtUpwdDnwd_Step1/7
  [DrvStFtUpwdDnwdPos] -> DrvSt_DrvStFtUpwdDnwd_Step1/3
  Drv_FtUpwdDnwdPosTrgt/1 -> DrvSt_DrvStFtUpwdDnwd_Step1/6, DrvSt_DrvStFtUpwdDnwd_Step1/5, DrvSt_DrvStFtUpwdDnwd_Step1/4
  [Step1En] -> DrvSt_DrvStFtUpwdDnwd_Step1/2
  [Trig] -> DrvSt_DrvStFtUpwdDnwd_Step1/1
  PA_KeSMSuModeReqDurgTm_Val/1 -> [Tick]
  Step1En/1 -> [Step1En]
  Mode_Trig/1 -> [Trig]
  Bus Selector1/1 -> [DrvStFtUpwdDnwdPosV]  "<IfVeSMSuDrvStFtUpwdDnwdPosV_Val_read>"
  Bus Selector/4 -> [DrvStCshnRrUpwdDnwdPos]  "<IfVeSMSuDrvStCshnRrUpwdDnwdPos_Val_read>"
  Bus Selector1/2 -> [DrvStBkReclnUpwdDnwdPosV]  "<IfVeSMSuDrvStBkReclnUpwdDnwdPosV_Val_read>"
  Bus Selector/2 -> [DrvStBkReclnUpwdDnwdPos]  "<IfVeSMSuDrvStBkReclnUpwdDnwdPos_Val_read>"
  Bus Selector/1 -> [DrvStFtUpwdDnwdPos]  "<IfVeSMSuDrvStFtUpwdDnwdPos_Val_read>"
  Bus Selector1/4 -> [DrvStCshnRrUpwdDnwdPosV]  "<IfVeSMSuDrvStCshnRrUpwdDnwdPosV_Val_read>"
  Bus Selector1/3 -> [DrvStCshnFrntUpwdDnwdPosV]  "<IfVeSMSuDrvStCshnFrntUpwdDnwdPosV_Val_read>"
  DrvCurPosV/1 -> Bus Selector1/1
  Bus Selector1/5 -> [DrvStFrwdBkwdPosV]  "<IfVeSMSuDrvStFrwdBkwdPosV_Val_read>"
  DrvCurPos/1 -> Bus Selector/1
  Bus Selector/3 -> [DrvStCshnFrntUpwdDnwdPos]  "<IfVeSMSuDrvStCshnFrntUpwdDnwdPos_Val_read>"
  Bus Selector/5 -> [DrvStFrwdBkwdPos]  "<IfVeSMSuDrvStFrwdBkwdPos_Val_read>"
  [Step1done_2] -> Unit Delay/1
  [FtUpwdDnwd_Step1_ini] -> DrvSt_Step1_ini/1
  PA_KeSMSwDltTrgtPos_Val14/1 -> Bus Creator/4  "DrvStLgrstUpwdDnwdTrgtPos"
  PA_KeSMSwDltTrgtPos_Val3/1 -> Bus Creator/5  "DrvStBkReclnUpwdDnwdTrgtPos"
  PA_KeSMSwDltTrgtPos_Val10/1 -> Bus Creator/1  "DrvStBlstOtwdInwdTrgtPos"
  PA_KeSMSwDltTrgtPos_Val16/1 -> Bus Creator/7  "DrvStCshnRrUpwdDnwdTrgtPos"
  PA_KeSMSwDltTrgtPos_Val13/1 -> Bus Creator/3  "DrvStHdrstUpwdDnwdTrgtPos"
  [DrvSt_FtUpwdDnwd_TarPos] -> Bus Creator/2  "DrvStFtUpwdDnwdTrgtPos"
  Bus Creator/1 -> Recv_DrvStTrgtPoss/1
  PA_KeSMSwDltTrgtPos_Val15/1 -> Bus Creator/6  "DrvStCshnFrntUpwdDnwdTrgtPos"
  PA_KeSMSwDltTrgtPos_Val2/1 -> Bus Creator/8  "DrvStFrwdBkwdTrgtPos"
  PA_KeSMSuMdMotFinshdTm_Val/1 -> [KeSMSuMdMotFinshdTm_Val]
  PA_KeSMSuFirstRwStFwdBkwdPosDelta_Val/1 -> [KeSMSuFirstRwStFwdBkwdPosDelta_Val]
  PA_KeSMSuFirstRwStFootrestPosDelta_Val/1 -> [KeSMSuFirstRwStFootrestPosDelta_Val]
  PA_KeSMSuFirstRwStBackPosDelta_Val/1 -> [KeSMSuFirstRwStBackPosDelta_Val]
  [KeSMSuMdMotFinshdTm_Val] -> DrvSt_DrvStFtUpwdDnwd_Step1/12
  Bus Selector2/1 -> [K_DrvStBkReclnUpwdDnwdPos]  "<BkReclnUpwdDnwdPos>"
  Bus Selector2/2 -> [K_DrvStBkReclnUpwdDnwdPosMax]  "<BkReclnUpwdDnwdPosMax>"
  Bus Selector2/3 -> [K_DrvStBkReclnUpwdDnwdPosMin]  "<BkReclnUpwdDnwdPosMin>"
  Bus Selector2/4 -> [K_DrvStFrwdBkwdPos]  "<FrwdBkwdPos>"
  Bus Selector2/5 -> [K_DrvStFrwdBkwdPosMax]  "<FrwdBkwdPosMax>"
  Bus Selector2/6 -> [K_DrvStFrwdBkwdPosMin]  "<FrwdBkwdPosMin>"
  Bus Selector2/7 -> [K_DrvStFtUpwdDnwdPos]  "<FtUpwdDnwdPos>"
  Bus Selector2/8 -> [K_DrvStFtUpwdDnwdPosMax]  "<FtUpwdDnwdPosMax>"
  Bus Selector2/9 -> [K_DrvStFtUpwdDnwdPosMin]  "<FtUpwdDnwdPosMin>"
  ModeStCalib_Drv/1 -> Bus Selector3/1
  Bus Selector3/1 -> Bus Selector2/1  "<VIPDrvSt>"
  PA_KeSMSwDltTrgtPos_Val5/1 -> DrvSt_DrvStFtUpwdDnwd_Step1/13
  StConfig/1 -> Bus Selector4/1
  Bus Selector4/1 -> [BkReclnUpwdDnwdMovConfig]  "<BkReclnUpwdDnwdMovConfig>"
  Bus Selector4/2 -> [FrwdBkwdMovConfig]  "<FrwdBkwdMovConfig>"
  Bus Selector4/3 -> [FtUpwdDnwdMovConfig]  "<FtUpwdDnwdMovConfig>"
  [FtUpwdDnwdMovConfig] -> DrvSt_DrvStFtUpwdDnwd_Step1/14
  PA_KeSMSwDltTrgtPos_Val7/1 -> IfVeSMSuDrvStRclCmdSrv_Val_writeRaw/1
  Logical Operator/1 -> DrvSt_Step1_done/1
  Unit Delay/1 -> Logical Operator/2
  [FtUpwdDnwd_Step1_ini] -> Logical Operator/1
  Relational Operator/1 -> Logical Operator10/2
  isSeatOccupied/1 -> Logical Operator10/1
  Logical Operator10/1 -> [ChildLocker]
  SecRwRtStChldLkRsp_L/1 -> Relational Operator/1
  PA_KeSMSwDltTrgtPos_Val4/1 -> Relational Operator/2
  [CntLow] -> DrvSt_DrvStFtUpwdDnwd_Step1/15
  PA_KeSMSuMdRetryTm1_Val/1 -> [CntLow]

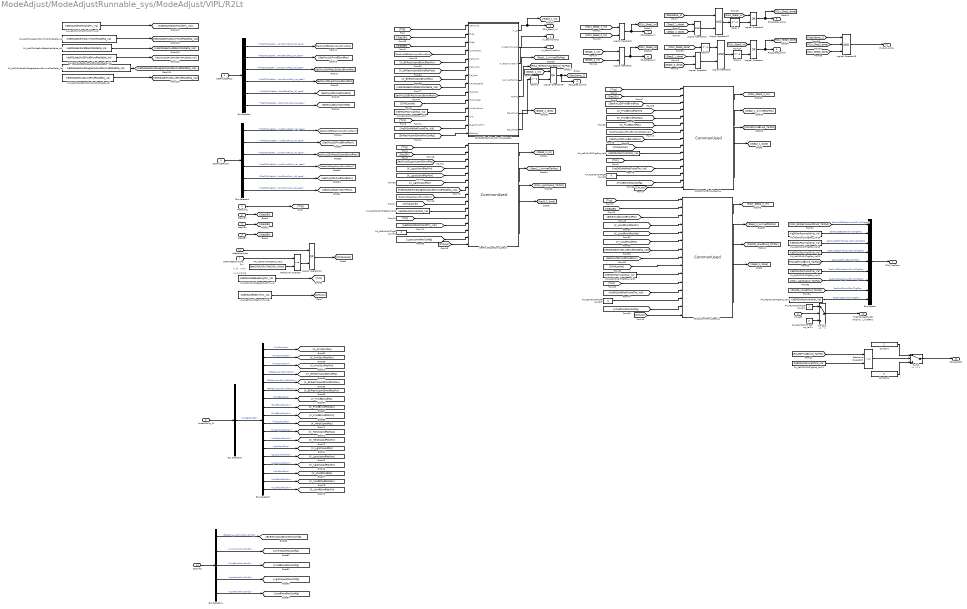
== system ModeAdjust/ModeAdjustRunnable_sys/ModeAdjust/VIPL/R2Lt ==
  note: %1锁，2未锁
  note: 2L 扶手屏位置
  Mode_Trig : Inport
  Step1En : Inport  Port=2
  Step2En : Inport  Port=3
  Step3En : Inport  Port=4
  SecRwLtStsPoss : Inport  Port=5
  SecRwLtStPossV : Inport  Port=6
  SecRwRtStChldLkRsp_L : Inport  Port=7
  VIP_Left : Inport  Port=8
  ModeStCalib_2L : Inport  Port=9
  StConfig : Inport  Port=10
  isSeatOccupied : Inport  Port=11
  Bus Creator : BusCreator  Inputs=9  OutDataTypeStr=Bus: SecRwLfSeatPos
  Bus Selector : BusSelector  OutputSignals=IfVeSMSuSecRwLtStBkReclnUpwdDnwdPos_Val_read,IfVeSMSuSecRwLtStFrwdBkwdPos_Val_read,IfVeSMSuSecRwLtStHPassStUpwdDnwdPos_Val_read,IfVeSMSuSecRwLtStLgrstUpwdDnwdPos_Val_read,IfVeSMSuSecRwLtStLtwdRtwdPos_Val_read,IfVeSMSuSecRwLtStArmScrnPos_Val_read
  Bus Selector1 : BusSelector  OutputSignals=IfVeSMSuSecRwLtStBkReclnUpwdDnwdPosV_Val_read,IfVeSMSuSecRwLtStFrwdBkwdPosV_Val_read,IfVeSMSuSecRwLtStHPassStUpwdDnwdPosV_Val_read,IfVeSMSuSecRwLtStLgrstUpwdDnwdPosV_Val_read,IfVeSMSuSecRwLtStLtwdRtwdPosV_Val_read,IfVeSMSuSecRwLtStArmScrnPosV_Val_read
  Bus Selector2 : BusSelector  OutputSignals=ArmScrnPos,ArmScrnPosMax,ArmScrnPosMin,BkReclnUpwdDnwdPos,BkReclnUpwdDnwdPosMax,BkReclnUpwdDnwdPosMin,FrwdBkwdPos,FrwdBkwdPosMax,FrwdBkwdPosMin,HdrstUpwdPos,HdrstUpwdPosMax,HdrstUpwdPosMin,LgrstUpwdPos,LgrstUpwdPosMax,LgrstUpwdPosMin,LtwdRtwdPos,LtwdRtwdPosMax,LtwdRtwdPosMin
  Bus Selector3 : BusSelector  OutputSignals=VIPSecRwLtSt
  Bus Selector4 : BusSelector  OutputSignals=BkReclnUpwdDnwdMovConfig,ArmTouchMovConfig,FrwdBkwdMovConfig,LgrstUpwdMovConfig,LtwdRtwdMovConfig
  Constant : Constant  Value=2  OutDataTypeStr=uint8
  Constant1 : Constant  Value=0  OutDataTypeStr=uint8
  Delay{1..4} (4 alike) : Delay  DelayLength=1
  Logical Operator{1..2,5..6,11..12} (6 alike) : Logic  AllPortsSameDT=off  OutDataTypeStr=boolean
  Logical Operator{3..4,10,16} (4 alike) : Logic  Operator=OR  AllPortsSameDT=off  OutDataTypeStr=boolean
  Logical Operator15 : Logic  Inputs=3  AllPortsSameDT=off  OutDataTypeStr=boolean
  PA_KeSMSuMdMotFinshdTm_Val : Constant  Value=KeSMSuMdMotFinshdTm_Val
  PA_KeSMSuMdRetryTm1_Val : Constant  Value=KeSMSuMdRetryTm1_Val
  PA_KeSMSuModeReqDurgTm_Val : Constant  Value=KeSMSuModeReqDurgTm_Val
  PA_KeSMSuSecRwStArmTochPosDelta_Val : Constant  Value=KeSMSuSecRwStArmTochPosDelta_Val
  PA_KeSMSuSecRwStBackPosDelta_Val : Constant  Value=KeSMSuSecRwStBackPosDelta_Val
  PA_KeSMSuSecRwStFwdBkwdPosDelta_Val : Constant  Value=KeSMSuSecRwStFwdBkwdPosDelta_Val
  PA_KeSMSuSecRwStLegrestUpwdDwnwdPosDelta_Val : Constant  Value=KeSMSuSecRwStLegrestUpwdDwnwdPosDelta_Val
  PA_KeSMSuSecRwStLwdRwdPosDelta_Val : Constant  Value=KeSMSuSecRwStLwdRwdPosDelta_Val
  PA_KeSMSwDltTrgtPos_Val{1,8..9,24} (4 alike) : Constant  Value=0  OutDataTypeStr=boolean
  PA_KeSMSwDltTrgtPos_Val{3,6..7,11..12,14,18..21} (10 alike) : Constant  Value=KeSMSwPosInvalidVal_Val
  PA_KeSMSwDltTrgtPos_Val2 : Constant  Value=SeatChldLkSt.ChldLkSt_Unlock
  PA_KeSMSwDltTrgtPos_Val4 : Constant  OutDataTypeStr=boolean
  R2LtSt_BkReclnUpwdDnwd_Lt_Step1 : Subsystem
  R2LtSt_FrwdBkwd_Step2_1 : Lib/CommonUsed  SystemSampleTime=-1
  R2LtSt_LtwdRtwd_Step2_2 : Lib/CommonUsed  SystemSampleTime=-1
  Relational Operator : RelationalOperator  Operator=~=  OutDataTypeStr=boolean  RndMeth=Simplest
  Relational Operator2 : RelationalOperator  Operator=~=  OutDataTypeStr=boolean  RndMeth=Simplest
  SecRwLtStLgrstUpwd_Step1 : Lib/CommonUsed  SystemSampleTime=-1
  Switch : Switch  Criteria=u2 ~= 0
  Switch2 : Switch  Criteria=u2 > Threshold
  R2Lt_Step1_Ini : Outport
  ini_ReclnOverUp : Outport  Port=2
  ini_ReclnOverDwn : Outport  Port=3
  R2Lt_Step2_Ini : Outport  Port=4
  R2Lt_Step1_done : Outport  Port=5
  R2Lt_Step2_done : Outport  Port=6
  R2Lt_TrgtPoss : Outport  Port=7  VectorParamsAs1DForOutWhenUnconnected=on
  R2Lt_Step3_Ini : Outport  Port=8
  R2Lt_Step3_done : Outport  Port=9
  IfVeSMSuSecRwLtStRclCmdSrv_Val_writeRaw : Outport  Port=10
  R2Lt_All_done : Outport  Port=11
  R2Lt_SpdCtrl : Outport  Port=12  VectorParamsAs1DForOutWhenUnconnected=on
  wires:
  Step2En/1 -> [Step2En]
  Step1En/1 -> [Step1En]
  PA_KeSMSwDltTrgtPos_Val20/1 -> Bus Creator/4  "SecRwLtStCshnRrUpwdDnwdTrgtPos"
  [R2LtStFrwdBkwd_TarPos] -> Bus Creator/5  "SecRwLtStFrwdBkwdTrgtPos"
  [R2Lt_BkReclnUpwdDnwd_TarPos] -> Bus Creator/1  "SecRwLtStBkReclnUpwdDnwdTrgtPos"
  PA_KeSMSwDltTrgtPos_Val18/1 -> Bus Creator/2  "SecRwLtStBlstOtwdInwdTrgtPos"
  [R2LtSt_LtwdRtwd_TarPos] -> Bus Creator/8  "SecRwLtStLtwdRtwdTrgtPos"
  PA_KeSMSwDltTrgtPos_Val19/1 -> Bus Creator/3  "SecRwLtStCshnFrntUpwdDnwdTrgtPos"
  [R2Lt_LgrstUpwd_TarPos] -> Bus Creator/7  "SecRwLtStLgrstUpwdDnwdTrgtPos"
  Bus Creator/1 -> R2Lt_TrgtPoss/1
  PA_KeSMSwDltTrgtPos_Val21/1 -> Bus Creator/6  "SecRwLtStHdrstUpwdDnwdTrgtPos"
  R2LtSt_LtwdRtwd_Step2_2/2 -> [Step2_2_ArrivedTarPos]
  R2LtSt_FrwdBkwd_Step2_1/2 -> [Step2_1_ArrivedTarPos]
  R2LtSt_BkReclnUpwdDnwd_Lt_Step1/6(Stg_done1) -> Delay3/1
  Logical Operator6/1 -> [R2Lt_Step2_Ini], R2Lt_Step2_Ini/1
  [R2Lt_Step2_2_ini] -> Logical Operator6/2
  [R2Lt_Step2_1_ini] -> Logical Operator6/1
  R2LtSt_BkReclnUpwdDnwd_Lt_Step1/1(ini_st) -> [Step3_1_ini], R2Lt_Step1_Ini/1
  [Step2En] -> R2LtSt_LtwdRtwd_Step2_2/2
  R2LtSt_LtwdRtwd_Step2_2/3 -> [R2LtSt_LtwdRtwd_TarPos]
  R2LtSt_LtwdRtwd_Step2_2/1 -> [R2Lt_Step2_2_ini]
  R2LtSt_LtwdRtwd_Step2_2/4 -> [Step2_2_done]
  [ChildLocker] -> R2LtSt_LtwdRtwd_Step2_2/9
  [KeSMSuSecRwStLwdRwdPosDelta_Val] -> R2LtSt_LtwdRtwd_Step2_2/7
  [Tick] -> R2LtSt_LtwdRtwd_Step2_2/11
  PA_KeSMSwDltTrgtPos_Val14/1 -> R2LtSt_LtwdRtwd_Step2_2/10
  [Trig] -> R2LtSt_LtwdRtwd_Step2_2/1
  [SecRwLtStLtwdRtwdPosV] -> R2LtSt_LtwdRtwd_Step2_2/8
  [SecRwLtStLtwdRtwdPos] -> R2LtSt_LtwdRtwd_Step2_2/3
  [K_LtwdRtwdPosMin] -> R2LtSt_LtwdRtwd_Step2_2/4
  SecRwLtStLgrstUpwd_Step1/4 -> [Step3_2_done]
  SecRwLtStLgrstUpwd_Step1/3 -> [R2Lt_LgrstUpwd_TarPos]
  SecRwLtStLgrstUpwd_Step1/2 -> [Step1_2_ArrivedTarPos]
  [Tick] -> SecRwLtStLgrstUpwd_Step1/11
  PA_KeSMSwDltTrgtPos_Val12/1 -> SecRwLtStLgrstUpwd_Step1/10
  [SecRwLtStLgrstUpwdDnwdPosV] -> SecRwLtStLgrstUpwd_Step1/8
  [KeSMSuSecRwStLegrestUpwdDwnwdPosDelta_Val] -> SecRwLtStLgrstUpwd_Step1/7
  [SecRwLtStBkReclnUpwdDnwdPosV] -> R2LtSt_BkReclnUpwdDnwd_Lt_Step1/9(PosValid)
  [SecRwLtStLgrstUpwdDnwdPos] -> SecRwLtStLgrstUpwd_Step1/3
  [Step3En] -> SecRwLtStLgrstUpwd_Step1/2
  [Trig] -> SecRwLtStLgrstUpwd_Step1/1
  PA_KeSMSwDltTrgtPos_Val2/1 -> Relational Operator/2
  SecRwRtStChldLkRsp_L/1 -> Relational Operator/1
  Bus Selector/1 -> [SecRwLtStBkReclnUpwdDnwdPos]  "<IfVeSMSuSecRwLtStBkReclnUpwdDnwdPos_Val_read>"
  Bus Selector1/2 -> [SecRwLtStFrwdBkwdPosV]  "<IfVeSMSuSecRwLtStFrwdBkwdPosV_Val_read>"
  Bus Selector1/1 -> [SecRwLtStBkReclnUpwdDnwdPosV]  "<IfVeSMSuSecRwLtStBkReclnUpwdDnwdPosV_Val_read>"
  Bus Selector/2 -> [SecRwLtStFrwdBkwdPos]  "<IfVeSMSuSecRwLtStFrwdBkwdPos_Val_read>"
  Bus Selector/4 -> [SecRwLtStLgrstUpwdDnwdPos]  "<IfVeSMSuSecRwLtStLgrstUpwdDnwdPos_Val_read>"
  Bus Selector1/5 -> [SecRwLtStLtwdRtwdPosV]  "<IfVeSMSuSecRwLtStLtwdRtwdPosV_Val_read>"
  Bus Selector/3 -> [SecRwLtStHPassStUpwdDnwdPos]  "<IfVeSMSuSecRwLtStHPassStUpwdDnwdPos_Val_read>"
  SecRwLtStPossV/1 -> Bus Selector1/1
  Bus Selector1/4 -> [SecRwLtStLgrstUpwdDnwdPosV]  "<IfVeSMSuSecRwLtStLgrstUpwdDnwdPosV_Val_read>"
  SecRwLtStsPoss/1 -> Bus Selector/1
  Bus Selector/5 -> [SecRwLtStLtwdRtwdPos]  "<IfVeSMSuSecRwLtStLtwdRtwdPos_Val_read>"
  Bus Selector1/3 -> [SecRwLtStHPassStUpwdDnwdPosV]  "<IfVeSMSuSecRwLtStHPassStUpwdDnwdPosV_Val_read>"
  R2LtSt_FrwdBkwd_Step2_1/4 -> [Step2_1_done]
  R2LtSt_FrwdBkwd_Step2_1/3 -> [R2LtStFrwdBkwd_TarPos]
  [Tick] -> R2LtSt_FrwdBkwd_Step2_1/11
  [Tick] -> R2LtSt_BkReclnUpwdDnwd_Lt_Step1/12(Tick)
  PA_KeSMSwDltTrgtPos_Val6/1 -> R2LtSt_FrwdBkwd_Step2_1/10
  [ChildLocker] -> R2LtSt_BkReclnUpwdDnwd_Lt_Step1/10(ChildLocker)
  [SecRwLtStFrwdBkwdPosV] -> R2LtSt_FrwdBkwd_Step2_1/8
  [K_FrwdBkwdPos] -> R2LtSt_FrwdBkwd_Step2_1/6
  [Step2En] -> R2LtSt_FrwdBkwd_Step2_1/2
  [Trig] -> R2LtSt_FrwdBkwd_Step2_1/1
  R2LtSt_BkReclnUpwdDnwd_Lt_Step1/5(TarPos) -> [R2Lt_BkReclnUpwdDnwd_TarPos]
  PA_KeSMSwDltTrgtPos_Val3/1 -> R2LtSt_BkReclnUpwdDnwd_Lt_Step1/11(InvalidValue)
  [K_BkReclnUpwdDnwdPos] -> R2LtSt_BkReclnUpwdDnwd_Lt_Step1/7(Tar_Pos)
  [SecRwLtStBkReclnUpwdDnwdPos] -> R2LtSt_BkReclnUpwdDnwd_Lt_Step1/4(Current_Pos)
  R2LtSt_BkReclnUpwdDnwd_Lt_Step1/4(isArrivedTarPos) -> [Step1_1_ArrivedTarPos]
  [K_BkReclnUpwdDnwdPosMin] -> R2LtSt_BkReclnUpwdDnwd_Lt_Step1/5(Calib_Min)
  R2LtSt_FrwdBkwd_Step2_1/1 -> [R2Lt_Step2_1_ini]
  [K_FrwdBkwdPosMin] -> R2LtSt_FrwdBkwd_Step2_1/4
  [KeSMSuSecRwStFwdBkwdPosDelta_Val] -> R2LtSt_FrwdBkwd_Step2_1/7
  [K_FrwdBkwdPosMax] -> R2LtSt_FrwdBkwd_Step2_1/5
  [SecRwLtStFrwdBkwdPos] -> R2LtSt_FrwdBkwd_Step2_1/3
  [KeSMSuSecRwStBackPosDelta_Val] -> R2LtSt_BkReclnUpwdDnwd_Lt_Step1/8(Tar_PosDelta)
  Mode_Trig/1 -> [Trig]
  [Trig] -> R2LtSt_BkReclnUpwdDnwd_Lt_Step1/1(MSM_Trig)
  [K_BkReclnUpwdDnwdPosMax] -> R2LtSt_BkReclnUpwdDnwd_Lt_Step1/6(Calib_Max)
  Step3En/1 -> [Step3En]
  [Step1En] -> R2LtSt_BkReclnUpwdDnwd_Lt_Step1/2(Ena1)
  [Step3En] -> R2LtSt_BkReclnUpwdDnwd_Lt_Step1/3(Ena3)
  [Step3_1_done] -> Logical Operator1/1
  [Step3_2_done] -> Logical Operator1/2
  Logical Operator2/1 -> [R2Lt_Step3_Ini], R2Lt_Step3_Ini/1
  SecRwLtStLgrstUpwd_Step1/1 -> [Step3_2_ini]
  [Step3_1_ini] -> Logical Operator2/1
  [Step3_2_ini] -> Logical Operator2/2
  R2LtSt_BkReclnUpwdDnwd_Lt_Step1/3(ini_ReclnOverDwn) -> ini_ReclnOverDwn/1
  R2LtSt_BkReclnUpwdDnwd_Lt_Step1/2(ini_ReclnOverUp) -> ini_ReclnOverUp/1
  Logical Operator5/1 -> Delay2/1
  [Step1done_1] -> Logical Operator12/1
  Logical Operator11/1 -> Logical Operator12/2
  Logical Operator1/1 -> Logical Operator5/2
  [Step2_2_done] -> Logical Operator11/2
  [R2Lt_Step2_done] -> Delay4/1
  Logical Operator12/1 -> Delay1/1
  [Step2_1_done] -> Logical Operator11/1
  Logical Operator3/1 -> [R2Lt_Step2_done], R2Lt_Step2_done/1
  Logical Operator16/1 -> [Step1done_1], R2Lt_Step1_done/1
  Delay1/1 -> Logical Operator3/2
  [R2Lt_Step2_Ini] -> Logical Operator3/1
  Delay2/1 -> Logical Operator4/2
  [R2Lt_Step3_Ini] -> Logical Operator4/1
  VIP_Left/1 -> Switch2/2
  PA_KeSMSwDltTrgtPos_Val4/1 -> Switch2/1
  PA_KeSMSwDltTrgtPos_Val24/1 -> Switch2/3
  Switch2/1 -> IfVeSMSuSecRwLtStRclCmdSrv_Val_writeRaw/1
  Logical Operator4/1 -> [R2Lt_Step3_done], R2Lt_Step3_done/1
  Delay3/1 -> Logical Operator16/2
  [Step3_1_ini] -> Logical Operator16/1
  [Step1done_1] -> Logical Operator15/1
  [R2Lt_Step2_done] -> Logical Operator15/2
  [R2Lt_Step3_done] -> Logical Operator15/3
  Logical Operator15/1 -> R2Lt_All_done/1
  [K_LgrstUpwdPosMin] -> SecRwLtStLgrstUpwd_Step1/4
  [K_LgrstUpwdPosMax] -> SecRwLtStLgrstUpwd_Step1/5
  [K_LgrstUpwdPos] -> SecRwLtStLgrstUpwd_Step1/6
  [K_LtwdRtwdPosMax] -> R2LtSt_LtwdRtwd_Step2_2/5
  [K_LtwdRtwdPos] -> R2LtSt_LtwdRtwd_Step2_2/6
  R2LtSt_BkReclnUpwdDnwd_Lt_Step1/7(Stg_done3) -> [Step3_1_done]
  PA_KeSMSwDltTrgtPos_Val7/1 -> Bus Creator/9  "SecRwLtStArmScrnTrgtPos"
  PA_KeSMSuSecRwStFwdBkwdPosDelta_Val/1 -> [KeSMSuSecRwStFwdBkwdPosDelta_Val]
  PA_KeSMSuSecRwStLegrestUpwdDwnwdPosDelta_Val/1 -> [KeSMSuSecRwStLegrestUpwdDwnwdPosDelta_Val]
  PA_KeSMSuSecRwStLwdRwdPosDelta_Val/1 -> [KeSMSuSecRwStLwdRwdPosDelta_Val]
  PA_KeSMSuSecRwStBackPosDelta_Val/1 -> [KeSMSuSecRwStBackPosDelta_Val]
  PA_KeSMSuMdMotFinshdTm_Val/1 -> [KeSMSuMdMotFinshdTm_Val]
  PA_KeSMSuSecRwStArmTochPosDelta_Val/1 -> [KeSMSuSecRwStArmTochPosDelta_Val]
  PA_KeSMSuModeReqDurgTm_Val/1 -> [Tick]
  [KeSMSuMdMotFinshdTm_Val] -> R2LtSt_BkReclnUpwdDnwd_Lt_Step1/13(CheckFinishTm)
  [KeSMSuMdMotFinshdTm_Val] -> SecRwLtStLgrstUpwd_Step1/12
  [KeSMSuMdMotFinshdTm_Val] -> R2LtSt_LtwdRtwd_Step2_2/12
  [KeSMSuMdMotFinshdTm_Val] -> R2LtSt_FrwdBkwd_Step2_1/12
  Bus Selector/6 -> [SecRwLtStArmScrnPos]  "<IfVeSMSuSecRwLtStArmScrnPos_Val_read>"
  Bus Selector1/6 -> [SecRwLtStArmScrnPosV]  "<IfVeSMSuSecRwLtStArmScrnPosV_Val_read>"
  Bus Selector2/1 -> [K_ArmScrnPos]  "<ArmScrnPos>"
  Bus Selector2/18 -> [K_LtwdRtwdPosMin]  "<LtwdRtwdPosMin>"
  Bus Selector2/16 -> [K_LtwdRtwdPos]  "<LtwdRtwdPos>"
  Bus Selector2/15 -> [K_LgrstUpwdPosMin]  "<LgrstUpwdPosMin>"
  Bus Selector2/17 -> [K_LtwdRtwdPosMax]  "<LtwdRtwdPosMax>"
  Bus Selector2/12 -> [K_HdrstUpwdPosMin]  "<HdrstUpwdPosMin>"
  Bus Selector2/13 -> [K_LgrstUpwdPos]  "<LgrstUpwdPos>"
  Bus Selector2/11 -> [K_HdrstUpwdPosMax]  "<HdrstUpwdPosMax>"
  Bus Selector2/14 -> [K_LgrstUpwdPosMax]  "<LgrstUpwdPosMax>"
  Bus Selector2/10 -> [K_HdrstUpwdPos]  "<HdrstUpwdPos>"
  Bus Selector2/4 -> [K_BkReclnUpwdDnwdPos]  "<BkReclnUpwdDnwdPos>"
  Bus Selector2/9 -> [K_FrwdBkwdPosMin]  "<FrwdBkwdPosMin>"
  Bus Selector2/5 -> [K_BkReclnUpwdDnwdPosMax]  "<BkReclnUpwdDnwdPosMax>"
  Bus Selector2/8 -> [K_FrwdBkwdPosMax]  "<FrwdBkwdPosMax>"
  Bus Selector3/1 -> Bus Selector2/1  "<VIPSecRwLtSt>"
  Bus Selector2/7 -> [K_FrwdBkwdPos]  "<FrwdBkwdPos>"
  Bus Selector2/3 -> [K_ArmScrnPosMin]  "<ArmScrnPosMin>"
  Bus Selector2/2 -> [K_ArmScrnPosMax]  "<ArmScrnPosMax>"
  Bus Selector2/6 -> [K_BkReclnUpwdDnwdPosMin]  "<BkReclnUpwdDnwdPosMin>"
  ModeStCalib_2L/1 -> Bus Selector3/1
  PA_KeSMSwDltTrgtPos_Val1/1 -> SecRwLtStLgrstUpwd_Step1/13
  PA_KeSMSwDltTrgtPos_Val8/1 -> R2LtSt_FrwdBkwd_Step2_1/13
  PA_KeSMSwDltTrgtPos_Val9/1 -> R2LtSt_LtwdRtwd_Step2_2/13
  Delay4/1 -> Logical Operator5/1
  Bus Selector4/5 -> [LtwdRtwdMovConfig]  "<LtwdRtwdMovConfig>"
  StConfig/1 -> Bus Selector4/1
  Bus Selector4/4 -> [LgrstUpwdMovConfig]  "<LgrstUpwdMovConfig>"
  Bus Selector4/1 -> [BkReclnUpwdDnwdMovConfig]  "<BkReclnUpwdDnwdMovConfig>"
  Bus Selector4/2 -> [ArmTouchMovConfig]  "<ArmTouchMovConfig>"
  Bus Selector4/3 -> [FrwdBkwdMovConfig]  "<FrwdBkwdMovConfig>"
  [BkReclnUpwdDnwdMovConfig] -> R2LtSt_BkReclnUpwdDnwd_Lt_Step1/14(StConfig)
  [LgrstUpwdMovConfig] -> SecRwLtStLgrstUpwd_Step1/14
  [FrwdBkwdMovConfig] -> R2LtSt_FrwdBkwd_Step2_1/14
  [LtwdRtwdMovConfig] -> R2LtSt_LtwdRtwd_Step2_2/14
  [ChildLocker] -> SecRwLtStLgrstUpwd_Step1/9
  [ChildLocker] -> R2LtSt_FrwdBkwd_Step2_1/9
  Relational Operator/1 -> Logical Operator10/2
  isSeatOccupied/1 -> Logical Operator10/1
  Logical Operator10/1 -> [ChildLocker]
  [CntLow] -> R2LtSt_FrwdBkwd_Step2_1/15
  [CntLow] -> R2LtSt_LtwdRtwd_Step2_2/15
  [CntLow] -> SecRwLtStLgrstUpwd_Step1/15
  PA_KeSMSuMdRetryTm1_Val/1 -> [CntLow]
  Switch/1 -> R2Lt_SpdCtrl/1
  Constant1/1 -> Switch/3
  [R2LtStFrwdBkwd_TarPos] -> Relational Operator2/1
  Relational Operator2/1 -> Switch/2
  PA_KeSMSwDltTrgtPos_Val11/1 -> Relational Operator2/2
  Constant/1 -> Switch/1
